simulink model "Tekercs_K6"  (R2025a)
settings: Solver=VariableStepAuto  StartTime=0.0  StopTime=250e-3  MaxStep=1e-3/25  RelTol=1e-3
settings Model: Creator=Szalay  LastModifiedBy=Szalay

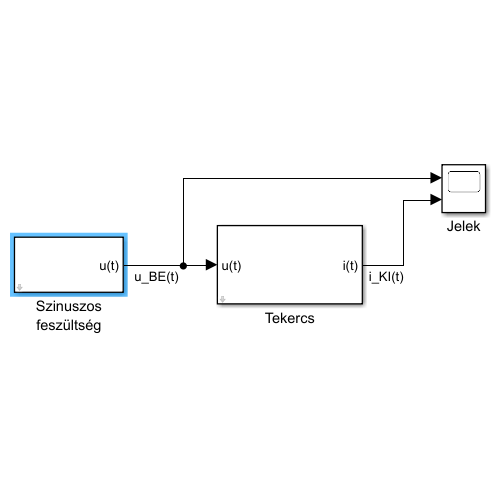
[thumbnail: Simulink's stored preview of the top-level diagram]
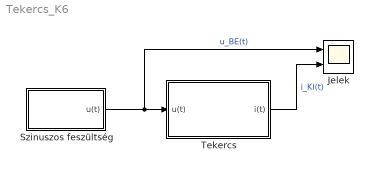
== system Tekercs_K6 ==
  Jelek : Scope  NumInputPorts=2
      settings: ActiveDisplayYMinimum=-1.2499999992410504  ActiveDisplayYMaximum=1.2499999999156723
  Szinuszos feszültség : Subsystem  mask(Szinuszos feszültségforrás){U_0=1, f=1/1e-3/(2*pi) / 10, q_0=0}
      mask prompts: U_0 "Amplitúdó"; f "Frekvencia (Hz)"; q_0 "Fáziseltolódás (rad)"
      mask help: Paraméterezhető feszültségforrás u(t) = U_0 cos(2 π f t + φ) alakban.
      mask DialogControl ParameterGroupVar Prompt: Beállítások
  Tekercs : Subsystem  mask(Tekercs){L=1e-3, R=1, i_0=0.5}
      mask prompts: L "Öninduktivitás (H)"; R "Ellenállás (Ohm)"; i_0 "Kezdeti áramerősség (A)"
      mask help: Lineáris mágnesezettségű tekercs modell (RL-tag).
      mask DialogControl ParameterGroupVar Prompt: Modellparaméterek
      mask DialogControl Container3 Prompt: Kezdeti érték
  wires:
  Tekercs/1(i(t)) -> Jelek/2  "i_KI(t)"
  Szinuszos feszültség/1(u(t)) -> Tekercs/1(u(t)), Jelek/1  "u_BE(t)"

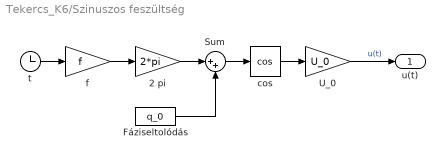
== system Tekercs_K6/Szinuszos feszültség ==
  2 pi : Gain  Gain=2*pi
  Fáziseltolódás : Constant  Value=q_0
  Sum : Sum  Inputs=|++
  U_0 : Gain  Gain=U_0
  cos : Trigonometry  Operator=cos
  f : Gain  Gain=f
  t : Clock
  u(t) : Outport
  wires:
  f/1 -> 2 pi/1
  U_0/1 -> u(t)/1  "u(t)"
  Fáziseltolódás/1 -> Sum/2
  2 pi/1 -> Sum/1
  Sum/1 -> cos/1
  t/1 -> f/1
  cos/1 -> U_0/1

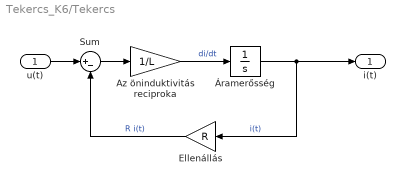
== system Tekercs_K6/Tekercs ==
  u(t) : Inport
  Az öninduktivitás reciproka : Gain  Gain=1/L
  Ellenállás : Gain  Gain=R
  Sum : Sum  Inputs=|+-
  Áramerősség : Integrator  InitialCondition=i_0
  i(t) : Outport
  wires:
  Áramerősség/1 -> i(t)/1, Ellenállás/1  "i(t)"
  Az öninduktivitás reciproka/1 -> Áramerősség/1  "di/dt"
  Ellenállás/1 -> Sum/2  "R i(t)"
  Sum/1 -> Az öninduktivitás reciproka/1
  u(t)/1 -> Sum/1
